simulink model "dcmotor_data"  (R2015a)
settings: Solver=ode23t  StartTime=0.0  StopTime=10.0  RelTol=1e-3  AbsTol=1e-3
libraries: fl_lib x104, nesl_utility x3, elec_lib x1
settings Model: Creator=sseshadr  LastModifiedBy=sseshadr
settings SimscapeCC: SimscapeLogType=all  SimscapeLogOpenViewer=on  SimscapeLogLimitData=off  SimscapeLogDataHistory=10000

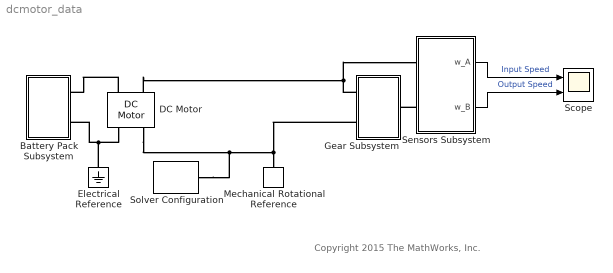
== system dcmotor_data ==
  note: Copyright 2015 The MathWorks, Inc.
  Battery Pack Subsystem : Subsystem
  DC Motor : elec_lib/Actuators & Drivers/Rotational Actuators/DC Motor  parameterization=1  Ra=0.0093 Ohm  La=172 uH  emf_or_torque=1  Kv=0.19 V/rpm  Ki=6.876e-4 N*m/A  T_stall=2.4e-4 N*m  w_max=1.91e+4 rpm  w_rated=1.5e+4 rpm  P_rated=0.08 W  V_rated=1.5 V  J=0.01 g*cm^2  lam_param=1  lam=0 N*m/(rad/s)  i_noload=0 A  V_i_noload=1.5 V  speed0=10 rad/s  alpha=0.00393 1/K  Tmeas=25 C  thermal_mass=100 J/K  initial_temperature=25 C
  Electrical Reference : fl_lib/Electrical/Electrical Elements/Electrical Reference
  Gear Subsystem : Subsystem
  Mechanical Rotational Reference : fl_lib/Mechanical/Rotational Elements/Mechanical Rotational Reference
  Scope : Scope  NumInputPorts=2
      settings: YMin=-5~-5  YMax=5~5
  Sensors Subsystem : Subsystem
  Solver Configuration : nesl_utility/Solver Configuration  PhysicalDomain=network_engine_domain  SubClassName=solver  LeftPortType=input  RightPortType=generic  Accelerate=off  Tones=[]  Harmonics=[]  SimulateNoise=off  Profile=off  UseLocalSampling=off  EnableSwitchedLinearOptims=on  FrequencyDomain=off  UseCCode=off  RelTol=0.001  AbsTol=1e-06  MinStep=1e-09  ToWorkspace=off  RevertToSquareIcSolve=off  NumHomotopyIterations=100  DoDC=off  ResidualTolerance=1e-09  UseLocalSolver=off  LocalSolverChoice=NE_BACKWARD_EULER_ADVANCER  LocalSolverSampleTime=0.001  DoFixedCost=off  MaxNonlinIter=3  MaxModeIter=2  LinearAlgebra=Sparse  DelaysMemoryBudget=1024  AutomaticFiltering=on  FilteringTimeConstant=0.001
  wires:
  Sensors Subsystem/1(w_A) -> Scope/1  "Input Speed"
  Sensors Subsystem/2(w_B) -> Scope/2  "Output Speed"
  connections:
  Solver Configuration/RConn1 -- DC Motor/RConn2 -- Gear Subsystem/LConn2 -- Mechanical Rotational Reference/LConn1
  Gear Subsystem/LConn1 -- DC Motor/LConn2 -- Sensors Subsystem/LConn1
  Sensors Subsystem/LConn2 -- Gear Subsystem/RConn1
  DC Motor/LConn1 -- Battery Pack Subsystem/RConn1
  DC Motor/RConn1 -- Electrical Reference/LConn1 -- Battery Pack Subsystem/RConn2

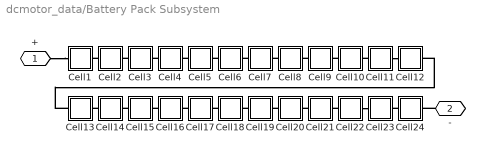
== system dcmotor_data/Battery Pack Subsystem ==
  Cell1 : Subsystem
  Cell10 : Subsystem
  Cell11 : Subsystem
  Cell12 : Subsystem
  Cell13 : Subsystem
  Cell14 : Subsystem
  Cell15 : Subsystem
  Cell16 : Subsystem
  Cell17 : Subsystem
  Cell18 : Subsystem
  Cell19 : Subsystem
  Cell2 : Subsystem
  Cell20 : Subsystem
  Cell21 : Subsystem
  Cell22 : Subsystem
  Cell23 : Subsystem
  Cell24 : Subsystem
  Cell3 : Subsystem
  Cell4 : Subsystem
  Cell5 : Subsystem
  Cell6 : Subsystem
  Cell7 : Subsystem
  Cell8 : Subsystem
  Cell9 : Subsystem
  + : PMIOPort  Port=1  Side=Right
  - : PMIOPort  Port=2  Side=Right
  connections:
  +/RConn1 -- Cell1/LConn1
  Cell2/LConn1 -- Cell1/RConn1
  Cell3/LConn1 -- Cell2/RConn1
  Cell4/LConn1 -- Cell3/RConn1
  Cell5/LConn1 -- Cell4/RConn1
  Cell6/LConn1 -- Cell5/RConn1
  Cell7/LConn1 -- Cell6/RConn1
  Cell8/LConn1 -- Cell7/RConn1
  Cell9/LConn1 -- Cell8/RConn1
  Cell10/LConn1 -- Cell9/RConn1
  Cell11/LConn1 -- Cell10/RConn1
  Cell13/LConn1 -- Cell12/RConn1
  Cell14/LConn1 -- Cell13/RConn1
  Cell15/LConn1 -- Cell14/RConn1
  Cell16/LConn1 -- Cell15/RConn1
  Cell17/LConn1 -- Cell16/RConn1
  Cell18/LConn1 -- Cell17/RConn1
  Cell19/LConn1 -- Cell18/RConn1
  Cell20/LConn1 -- Cell19/RConn1
  Cell21/LConn1 -- Cell20/RConn1
  Cell22/LConn1 -- Cell21/RConn1
  Cell24/LConn1 -- Cell23/RConn1
  -/RConn1 -- Cell24/RConn1
  Cell11/RConn1 -- Cell12/LConn1
  Cell22/RConn1 -- Cell23/LConn1

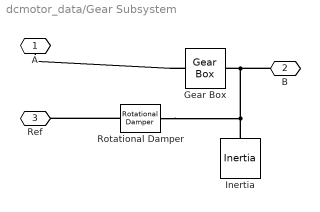
== system dcmotor_data/Gear Subsystem ==
  Gear Box : fl_lib/Mechanical/Mechanisms/Gear Box  ratio=2  t_in_specify=off  t_in_priority=High  t_in=0 N*m  t_out_specify=off  t_out_priority=High  t_out=0 N*m
  Inertia : fl_lib/Mechanical/Rotational Elements/Inertia  inertia=0.01 kg*m^2  w_specify=on  w_priority=Low  w=10 rad/s  t_specify=off  t_priority=High  t=0 N*m
  Rotational Damper : fl_lib/Mechanical/Rotational Elements/Rotational Damper  D=0.001 N*m/(rad/s)  w_specify=off  w_priority=High  w=0 rad/s  t_specify=off  t_priority=High  t=0 N*m
  A : PMIOPort  Port=1  Side=Left
  B : PMIOPort  Port=2  Side=Right
  Ref : PMIOPort  Port=3  Side=Left
  connections:
  Inertia/LConn1 -- Rotational Damper/LConn1 -- B/RConn1 -- Gear Box/RConn1
  Rotational Damper/RConn1 -- Ref/RConn1
  Gear Box/LConn1 -- A/RConn1

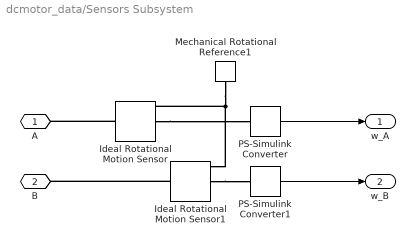
== system dcmotor_data/Sensors Subsystem ==
  Ideal Rotational Motion Sensor : fl_lib/Mechanical/Mechanical Sensors/Ideal Rotational Motion Sensor  offset=0 rad
  Ideal Rotational Motion Sensor1 : fl_lib/Mechanical/Mechanical Sensors/Ideal Rotational Motion Sensor  offset=0 rad
  Mechanical Rotational Reference1 : fl_lib/Mechanical/Rotational Elements/Mechanical Rotational Reference
  PS-Simulink Converter : nesl_utility/PS-Simulink Converter  PhysicalDomain=network_engine_domain  SubClassName=ps_output  LeftPortType=input  RightPortType=output  PseudoPeriodic=off  Frequencies=[]  Unit=1  AffineConversion=off
  PS-Simulink Converter1 : nesl_utility/PS-Simulink Converter  PhysicalDomain=network_engine_domain  SubClassName=ps_output  LeftPortType=input  RightPortType=output  PseudoPeriodic=off  Frequencies=[]  Unit=1  AffineConversion=off
  A : PMIOPort  Port=1  Side=Left
  B : PMIOPort  Port=2  Side=Left
  w_A : Outport
  w_B : Outport  Port=2
  wires:
  PS-Simulink Converter1/1 -> w_B/1
  PS-Simulink Converter/1 -> w_A/1
  connections:
  Ideal Rotational Motion Sensor/LConn1 -- A/RConn1
  Ideal Rotational Motion Sensor1/RConn2 -- PS-Simulink Converter1/LConn1
  Ideal Rotational Motion Sensor/RConn2 -- PS-Simulink Converter/LConn1
  Mechanical Rotational Reference1/LConn1 -- Ideal Rotational Motion Sensor/RConn1 -- Ideal Rotational Motion Sensor1/RConn1
  Ideal Rotational Motion Sensor1/LConn1 -- B/RConn1

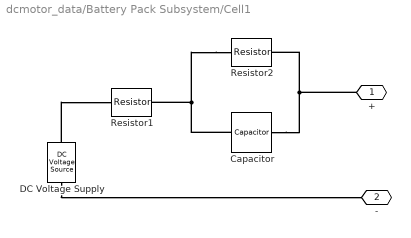
== system dcmotor_data/Battery Pack Subsystem/Cell1 ==
  Capacitor : fl_lib/Electrical/Electrical Elements/Capacitor  c=1e-3 F  r=1e-6 Ohm  g=0 1/Ohm  i_specify=off  i_priority=High  i=0 A  v_specify=off  v_priority=High  v=0 V  vc_specify=on  vc_priority=High  vc=0 V
  DC Voltage Supply : fl_lib/Electrical/Electrical Sources/DC Voltage Source  v0=4.2 V
  Resistor1 : fl_lib/Electrical/Electrical Elements/Resistor  R=0.07 Ohm  i_specify=off  i_priority=High  i=0 A  v_specify=off  v_priority=High  v=0 V
  Resistor2 : fl_lib/Electrical/Electrical Elements/Resistor  R=0.05 Ohm  i_specify=off  i_priority=High  i=0 A  v_specify=off  v_priority=High  v=0 V
  + : PMIOPort  Port=1  Side=Left
  - : PMIOPort  Port=2  Side=Right
  connections:
  Resistor2/LConn1 -- Capacitor/LConn1 -- Resistor1/RConn1
  DC Voltage Supply/RConn1 -- -/RConn1
  Resistor2/RConn1 -- +/RConn1 -- Capacitor/RConn1
  DC Voltage Supply/LConn1 -- Resistor1/LConn1

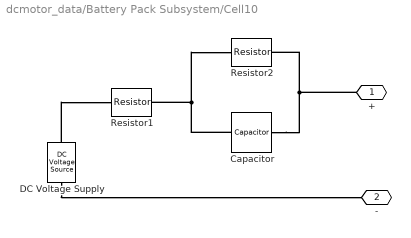
== system dcmotor_data/Battery Pack Subsystem/Cell10 ==
  Capacitor : fl_lib/Electrical/Electrical Elements/Capacitor  c=1e-3 F  r=1e-6 Ohm  g=0 1/Ohm  i_specify=off  i_priority=High  i=0 A  v_specify=off  v_priority=High  v=0 V  vc_specify=on  vc_priority=High  vc=0 V
  DC Voltage Supply : fl_lib/Electrical/Electrical Sources/DC Voltage Source  v0=4.2 V
  Resistor1 : fl_lib/Electrical/Electrical Elements/Resistor  R=0.07 Ohm  i_specify=off  i_priority=High  i=0 A  v_specify=off  v_priority=High  v=0 V
  Resistor2 : fl_lib/Electrical/Electrical Elements/Resistor  R=0.05 Ohm  i_specify=off  i_priority=High  i=0 A  v_specify=off  v_priority=High  v=0 V
  + : PMIOPort  Port=1  Side=Left
  - : PMIOPort  Port=2  Side=Right
  connections:
  DC Voltage Supply/LConn1 -- Resistor1/LConn1
  +/RConn1 -- Capacitor/RConn1 -- Resistor2/RConn1
  DC Voltage Supply/RConn1 -- -/RConn1
  Resistor1/RConn1 -- Capacitor/LConn1 -- Resistor2/LConn1

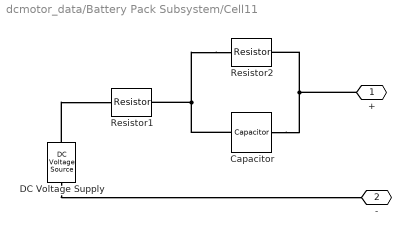
== system dcmotor_data/Battery Pack Subsystem/Cell11 ==
  Capacitor : fl_lib/Electrical/Electrical Elements/Capacitor  c=1e-3 F  r=1e-6 Ohm  g=0 1/Ohm  i_specify=off  i_priority=High  i=0 A  v_specify=off  v_priority=High  v=0 V  vc_specify=on  vc_priority=High  vc=0 V
  DC Voltage Supply : fl_lib/Electrical/Electrical Sources/DC Voltage Source  v0=4.2 V
  Resistor1 : fl_lib/Electrical/Electrical Elements/Resistor  R=0.07 Ohm  i_specify=off  i_priority=High  i=0 A  v_specify=off  v_priority=High  v=0 V
  Resistor2 : fl_lib/Electrical/Electrical Elements/Resistor  R=0.05 Ohm  i_specify=off  i_priority=High  i=0 A  v_specify=off  v_priority=High  v=0 V
  + : PMIOPort  Port=1  Side=Left
  - : PMIOPort  Port=2  Side=Right
  connections:
  Resistor2/LConn1 -- Capacitor/LConn1 -- Resistor1/RConn1
  DC Voltage Supply/RConn1 -- -/RConn1
  Resistor2/RConn1 -- Capacitor/RConn1 -- +/RConn1
  DC Voltage Supply/LConn1 -- Resistor1/LConn1

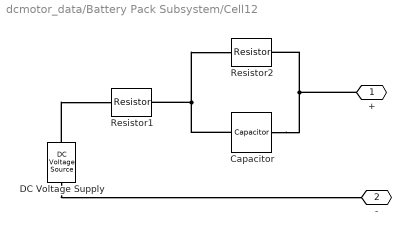
== system dcmotor_data/Battery Pack Subsystem/Cell12 ==
  Capacitor : fl_lib/Electrical/Electrical Elements/Capacitor  c=1e-3 F  r=1e-6 Ohm  g=0 1/Ohm  i_specify=off  i_priority=High  i=0 A  v_specify=off  v_priority=High  v=0 V  vc_specify=on  vc_priority=High  vc=0 V
  DC Voltage Supply : fl_lib/Electrical/Electrical Sources/DC Voltage Source  v0=4.2 V
  Resistor1 : fl_lib/Electrical/Electrical Elements/Resistor  R=0.07 Ohm  i_specify=off  i_priority=High  i=0 A  v_specify=off  v_priority=High  v=0 V
  Resistor2 : fl_lib/Electrical/Electrical Elements/Resistor  R=0.05 Ohm  i_specify=off  i_priority=High  i=0 A  v_specify=off  v_priority=High  v=0 V
  + : PMIOPort  Port=1  Side=Left
  - : PMIOPort  Port=2  Side=Right
  connections:
  DC Voltage Supply/LConn1 -- Resistor1/LConn1
  +/RConn1 -- Capacitor/RConn1 -- Resistor2/RConn1
  DC Voltage Supply/RConn1 -- -/RConn1
  Resistor1/RConn1 -- Capacitor/LConn1 -- Resistor2/LConn1

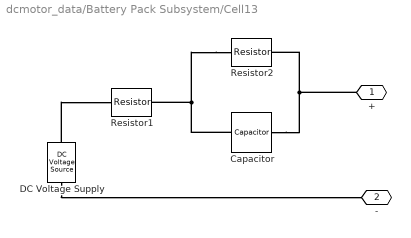
== system dcmotor_data/Battery Pack Subsystem/Cell13 ==
  Capacitor : fl_lib/Electrical/Electrical Elements/Capacitor  c=1e-3 F  r=1e-6 Ohm  g=0 1/Ohm  i_specify=off  i_priority=High  i=0 A  v_specify=off  v_priority=High  v=0 V  vc_specify=on  vc_priority=High  vc=0 V
  DC Voltage Supply : fl_lib/Electrical/Electrical Sources/DC Voltage Source  v0=4.2 V
  Resistor1 : fl_lib/Electrical/Electrical Elements/Resistor  R=0.07 Ohm  i_specify=off  i_priority=High  i=0 A  v_specify=off  v_priority=High  v=0 V
  Resistor2 : fl_lib/Electrical/Electrical Elements/Resistor  R=0.05 Ohm  i_specify=off  i_priority=High  i=0 A  v_specify=off  v_priority=High  v=0 V
  + : PMIOPort  Port=1  Side=Left
  - : PMIOPort  Port=2  Side=Right
  connections:
  Resistor2/LConn1 -- Capacitor/LConn1 -- Resistor1/RConn1
  DC Voltage Supply/RConn1 -- -/RConn1
  Resistor2/RConn1 -- Capacitor/RConn1 -- +/RConn1
  DC Voltage Supply/LConn1 -- Resistor1/LConn1

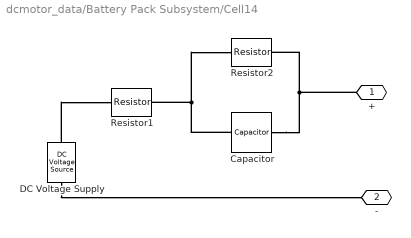
== system dcmotor_data/Battery Pack Subsystem/Cell14 ==
  Capacitor : fl_lib/Electrical/Electrical Elements/Capacitor  c=1e-3 F  r=1e-6 Ohm  g=0 1/Ohm  i_specify=off  i_priority=High  i=0 A  v_specify=off  v_priority=High  v=0 V  vc_specify=on  vc_priority=High  vc=0 V
  DC Voltage Supply : fl_lib/Electrical/Electrical Sources/DC Voltage Source  v0=4.2 V
  Resistor1 : fl_lib/Electrical/Electrical Elements/Resistor  R=0.07 Ohm  i_specify=off  i_priority=High  i=0 A  v_specify=off  v_priority=High  v=0 V
  Resistor2 : fl_lib/Electrical/Electrical Elements/Resistor  R=0.05 Ohm  i_specify=off  i_priority=High  i=0 A  v_specify=off  v_priority=High  v=0 V
  + : PMIOPort  Port=1  Side=Left
  - : PMIOPort  Port=2  Side=Right
  connections:
  DC Voltage Supply/LConn1 -- Resistor1/LConn1
  +/RConn1 -- Capacitor/RConn1 -- Resistor2/RConn1
  DC Voltage Supply/RConn1 -- -/RConn1
  Resistor1/RConn1 -- Capacitor/LConn1 -- Resistor2/LConn1

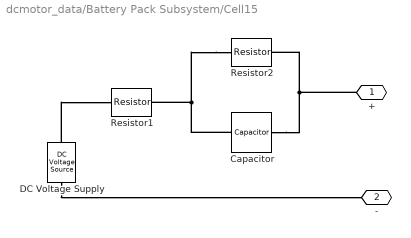
== system dcmotor_data/Battery Pack Subsystem/Cell15 ==
  Capacitor : fl_lib/Electrical/Electrical Elements/Capacitor  c=1e-3 F  r=1e-6 Ohm  g=0 1/Ohm  i_specify=off  i_priority=High  i=0 A  v_specify=off  v_priority=High  v=0 V  vc_specify=on  vc_priority=High  vc=0 V
  DC Voltage Supply : fl_lib/Electrical/Electrical Sources/DC Voltage Source  v0=4.2 V
  Resistor1 : fl_lib/Electrical/Electrical Elements/Resistor  R=0.07 Ohm  i_specify=off  i_priority=High  i=0 A  v_specify=off  v_priority=High  v=0 V
  Resistor2 : fl_lib/Electrical/Electrical Elements/Resistor  R=0.05 Ohm  i_specify=off  i_priority=High  i=0 A  v_specify=off  v_priority=High  v=0 V
  + : PMIOPort  Port=1  Side=Left
  - : PMIOPort  Port=2  Side=Right
  connections:
  Resistor2/LConn1 -- Capacitor/LConn1 -- Resistor1/RConn1
  DC Voltage Supply/RConn1 -- -/RConn1
  Resistor2/RConn1 -- Capacitor/RConn1 -- +/RConn1
  DC Voltage Supply/LConn1 -- Resistor1/LConn1

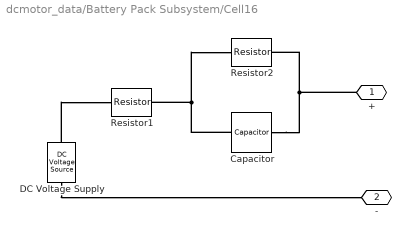
== system dcmotor_data/Battery Pack Subsystem/Cell16 ==
  Capacitor : fl_lib/Electrical/Electrical Elements/Capacitor  c=1e-3 F  r=1e-6 Ohm  g=0 1/Ohm  i_specify=off  i_priority=High  i=0 A  v_specify=off  v_priority=High  v=0 V  vc_specify=on  vc_priority=High  vc=0 V
  DC Voltage Supply : fl_lib/Electrical/Electrical Sources/DC Voltage Source  v0=4.2 V
  Resistor1 : fl_lib/Electrical/Electrical Elements/Resistor  R=0.07 Ohm  i_specify=off  i_priority=High  i=0 A  v_specify=off  v_priority=High  v=0 V
  Resistor2 : fl_lib/Electrical/Electrical Elements/Resistor  R=0.05 Ohm  i_specify=off  i_priority=High  i=0 A  v_specify=off  v_priority=High  v=0 V
  + : PMIOPort  Port=1  Side=Left
  - : PMIOPort  Port=2  Side=Right
  connections:
  DC Voltage Supply/LConn1 -- Resistor1/LConn1
  +/RConn1 -- Capacitor/RConn1 -- Resistor2/RConn1
  DC Voltage Supply/RConn1 -- -/RConn1
  Resistor1/RConn1 -- Capacitor/LConn1 -- Resistor2/LConn1

== system dcmotor_data/Battery Pack Subsystem/Cell17 ==
  Capacitor : fl_lib/Electrical/Electrical Elements/Capacitor  c=1e-3 F  r=1e-6 Ohm  g=0 1/Ohm  i_specify=off  i_priority=High  i=0 A  v_specify=off  v_priority=High  v=0 V  vc_specify=on  vc_priority=High  vc=0 V
  DC Voltage Supply : fl_lib/Electrical/Electrical Sources/DC Voltage Source  v0=4.2 V
  Resistor1 : fl_lib/Electrical/Electrical Elements/Resistor  R=0.07 Ohm  i_specify=off  i_priority=High  i=0 A  v_specify=off  v_priority=High  v=0 V
  Resistor2 : fl_lib/Electrical/Electrical Elements/Resistor  R=0.05 Ohm  i_specify=off  i_priority=High  i=0 A  v_specify=off  v_priority=High  v=0 V
  + : PMIOPort  Port=1  Side=Left
  - : PMIOPort  Port=2  Side=Right
  connections:
  Resistor2/LConn1 -- Capacitor/LConn1 -- Resistor1/RConn1
  DC Voltage Supply/RConn1 -- -/RConn1
  Resistor2/RConn1 -- Capacitor/RConn1 -- +/RConn1
  DC Voltage Supply/LConn1 -- Resistor1/LConn1

== system dcmotor_data/Battery Pack Subsystem/Cell18 ==
  Capacitor : fl_lib/Electrical/Electrical Elements/Capacitor  c=1e-3 F  r=1e-6 Ohm  g=0 1/Ohm  i_specify=off  i_priority=High  i=0 A  v_specify=off  v_priority=High  v=0 V  vc_specify=on  vc_priority=High  vc=0 V
  DC Voltage Supply : fl_lib/Electrical/Electrical Sources/DC Voltage Source  v0=4.2 V
  Resistor1 : fl_lib/Electrical/Electrical Elements/Resistor  R=0.07 Ohm  i_specify=off  i_priority=High  i=0 A  v_specify=off  v_priority=High  v=0 V
  Resistor2 : fl_lib/Electrical/Electrical Elements/Resistor  R=0.05 Ohm  i_specify=off  i_priority=High  i=0 A  v_specify=off  v_priority=High  v=0 V
  + : PMIOPort  Port=1  Side=Left
  - : PMIOPort  Port=2  Side=Right
  connections:
  DC Voltage Supply/LConn1 -- Resistor1/LConn1
  +/RConn1 -- Capacitor/RConn1 -- Resistor2/RConn1
  DC Voltage Supply/RConn1 -- -/RConn1
  Resistor1/RConn1 -- Capacitor/LConn1 -- Resistor2/LConn1

== system dcmotor_data/Battery Pack Subsystem/Cell19 ==
  Capacitor : fl_lib/Electrical/Electrical Elements/Capacitor  c=1e-3 F  r=1e-6 Ohm  g=0 1/Ohm  i_specify=off  i_priority=High  i=0 A  v_specify=off  v_priority=High  v=0 V  vc_specify=on  vc_priority=High  vc=0 V
  DC Voltage Supply : fl_lib/Electrical/Electrical Sources/DC Voltage Source  v0=4.2 V
  Resistor1 : fl_lib/Electrical/Electrical Elements/Resistor  R=0.07 Ohm  i_specify=off  i_priority=High  i=0 A  v_specify=off  v_priority=High  v=0 V
  Resistor2 : fl_lib/Electrical/Electrical Elements/Resistor  R=0.05 Ohm  i_specify=off  i_priority=High  i=0 A  v_specify=off  v_priority=High  v=0 V
  + : PMIOPort  Port=1  Side=Left
  - : PMIOPort  Port=2  Side=Right
  connections:
  Resistor2/LConn1 -- Capacitor/LConn1 -- Resistor1/RConn1
  DC Voltage Supply/RConn1 -- -/RConn1
  Resistor2/RConn1 -- Capacitor/RConn1 -- +/RConn1
  DC Voltage Supply/LConn1 -- Resistor1/LConn1

== system dcmotor_data/Battery Pack Subsystem/Cell2 ==
  Capacitor : fl_lib/Electrical/Electrical Elements/Capacitor  c=1e-3 F  r=1e-6 Ohm  g=0 1/Ohm  i_specify=off  i_priority=High  i=0 A  v_specify=off  v_priority=High  v=0 V  vc_specify=on  vc_priority=High  vc=0 V
  DC Voltage Supply : fl_lib/Electrical/Electrical Sources/DC Voltage Source  v0=4.2 V
  Resistor1 : fl_lib/Electrical/Electrical Elements/Resistor  R=0.07 Ohm  i_specify=off  i_priority=High  i=0 A  v_specify=off  v_priority=High  v=0 V
  Resistor2 : fl_lib/Electrical/Electrical Elements/Resistor  R=0.05 Ohm  i_specify=off  i_priority=High  i=0 A  v_specify=off  v_priority=High  v=0 V
  + : PMIOPort  Port=1  Side=Left
  - : PMIOPort  Port=2  Side=Right
  connections:
  DC Voltage Supply/LConn1 -- Resistor1/LConn1
  +/RConn1 -- Capacitor/RConn1 -- Resistor2/RConn1
  DC Voltage Supply/RConn1 -- -/RConn1
  Resistor1/RConn1 -- Capacitor/LConn1 -- Resistor2/LConn1

== system dcmotor_data/Battery Pack Subsystem/Cell20 ==
  Capacitor : fl_lib/Electrical/Electrical Elements/Capacitor  c=1e-3 F  r=1e-6 Ohm  g=0 1/Ohm  i_specify=off  i_priority=High  i=0 A  v_specify=off  v_priority=High  v=0 V  vc_specify=on  vc_priority=High  vc=0 V
  DC Voltage Supply : fl_lib/Electrical/Electrical Sources/DC Voltage Source  v0=4.2 V
  Resistor1 : fl_lib/Electrical/Electrical Elements/Resistor  R=0.07 Ohm  i_specify=off  i_priority=High  i=0 A  v_specify=off  v_priority=High  v=0 V
  Resistor2 : fl_lib/Electrical/Electrical Elements/Resistor  R=0.05 Ohm  i_specify=off  i_priority=High  i=0 A  v_specify=off  v_priority=High  v=0 V
  + : PMIOPort  Port=1  Side=Left
  - : PMIOPort  Port=2  Side=Right
  connections:
  DC Voltage Supply/LConn1 -- Resistor1/LConn1
  +/RConn1 -- Capacitor/RConn1 -- Resistor2/RConn1
  DC Voltage Supply/RConn1 -- -/RConn1
  Resistor1/RConn1 -- Capacitor/LConn1 -- Resistor2/LConn1

== system dcmotor_data/Battery Pack Subsystem/Cell21 ==
  Capacitor : fl_lib/Electrical/Electrical Elements/Capacitor  c=1e-3 F  r=1e-6 Ohm  g=0 1/Ohm  i_specify=off  i_priority=High  i=0 A  v_specify=off  v_priority=High  v=0 V  vc_specify=on  vc_priority=High  vc=0 V
  DC Voltage Supply : fl_lib/Electrical/Electrical Sources/DC Voltage Source  v0=4.2 V
  Resistor1 : fl_lib/Electrical/Electrical Elements/Resistor  R=0.07 Ohm  i_specify=off  i_priority=High  i=0 A  v_specify=off  v_priority=High  v=0 V
  Resistor2 : fl_lib/Electrical/Electrical Elements/Resistor  R=0.05 Ohm  i_specify=off  i_priority=High  i=0 A  v_specify=off  v_priority=High  v=0 V
  + : PMIOPort  Port=1  Side=Left
  - : PMIOPort  Port=2  Side=Right
  connections:
  Resistor2/LConn1 -- Capacitor/LConn1 -- Resistor1/RConn1
  DC Voltage Supply/RConn1 -- -/RConn1
  Resistor2/RConn1 -- Capacitor/RConn1 -- +/RConn1
  DC Voltage Supply/LConn1 -- Resistor1/LConn1

== system dcmotor_data/Battery Pack Subsystem/Cell22 ==
  Capacitor : fl_lib/Electrical/Electrical Elements/Capacitor  c=1e-3 F  r=1e-6 Ohm  g=0 1/Ohm  i_specify=off  i_priority=High  i=0 A  v_specify=off  v_priority=High  v=0 V  vc_specify=on  vc_priority=High  vc=0 V
  DC Voltage Supply : fl_lib/Electrical/Electrical Sources/DC Voltage Source  v0=4.2 V
  Resistor1 : fl_lib/Electrical/Electrical Elements/Resistor  R=0.07 Ohm  i_specify=off  i_priority=High  i=0 A  v_specify=off  v_priority=High  v=0 V
  Resistor2 : fl_lib/Electrical/Electrical Elements/Resistor  R=0.05 Ohm  i_specify=off  i_priority=High  i=0 A  v_specify=off  v_priority=High  v=0 V
  + : PMIOPort  Port=1  Side=Left
  - : PMIOPort  Port=2  Side=Right
  connections:
  DC Voltage Supply/LConn1 -- Resistor1/LConn1
  +/RConn1 -- Capacitor/RConn1 -- Resistor2/RConn1
  DC Voltage Supply/RConn1 -- -/RConn1
  Resistor1/RConn1 -- Capacitor/LConn1 -- Resistor2/LConn1

== system dcmotor_data/Battery Pack Subsystem/Cell23 ==
  Capacitor : fl_lib/Electrical/Electrical Elements/Capacitor  c=1e-3 F  r=1e-6 Ohm  g=0 1/Ohm  i_specify=off  i_priority=High  i=0 A  v_specify=off  v_priority=High  v=0 V  vc_specify=on  vc_priority=High  vc=0 V
  DC Voltage Supply : fl_lib/Electrical/Electrical Sources/DC Voltage Source  v0=4.2 V
  Resistor1 : fl_lib/Electrical/Electrical Elements/Resistor  R=0.07 Ohm  i_specify=off  i_priority=High  i=0 A  v_specify=off  v_priority=High  v=0 V
  Resistor2 : fl_lib/Electrical/Electrical Elements/Resistor  R=0.05 Ohm  i_specify=off  i_priority=High  i=0 A  v_specify=off  v_priority=High  v=0 V
  + : PMIOPort  Port=1  Side=Left
  - : PMIOPort  Port=2  Side=Right
  connections:
  Resistor2/LConn1 -- Capacitor/LConn1 -- Resistor1/RConn1
  DC Voltage Supply/RConn1 -- -/RConn1
  Resistor2/RConn1 -- Capacitor/RConn1 -- +/RConn1
  DC Voltage Supply/LConn1 -- Resistor1/LConn1

== system dcmotor_data/Battery Pack Subsystem/Cell24 ==
  Capacitor : fl_lib/Electrical/Electrical Elements/Capacitor  c=1e-3 F  r=1e-6 Ohm  g=0 1/Ohm  i_specify=off  i_priority=High  i=0 A  v_specify=off  v_priority=High  v=0 V  vc_specify=on  vc_priority=High  vc=0 V
  DC Voltage Supply : fl_lib/Electrical/Electrical Sources/DC Voltage Source  v0=4.2 V
  Resistor1 : fl_lib/Electrical/Electrical Elements/Resistor  R=0.07 Ohm  i_specify=off  i_priority=High  i=0 A  v_specify=off  v_priority=High  v=0 V
  Resistor2 : fl_lib/Electrical/Electrical Elements/Resistor  R=0.05 Ohm  i_specify=off  i_priority=High  i=0 A  v_specify=off  v_priority=High  v=0 V
  + : PMIOPort  Port=1  Side=Left
  - : PMIOPort  Port=2  Side=Right
  connections:
  DC Voltage Supply/LConn1 -- Resistor1/LConn1
  +/RConn1 -- Capacitor/RConn1 -- Resistor2/RConn1
  DC Voltage Supply/RConn1 -- -/RConn1
  Resistor1/RConn1 -- Capacitor/LConn1 -- Resistor2/LConn1

== system dcmotor_data/Battery Pack Subsystem/Cell3 ==
  Capacitor : fl_lib/Electrical/Electrical Elements/Capacitor  c=1e-3 F  r=1e-6 Ohm  g=0 1/Ohm  i_specify=off  i_priority=High  i=0 A  v_specify=off  v_priority=High  v=0 V  vc_specify=on  vc_priority=High  vc=0 V
  DC Voltage Supply : fl_lib/Electrical/Electrical Sources/DC Voltage Source  v0=4.2 V
  Resistor1 : fl_lib/Electrical/Electrical Elements/Resistor  R=0.07 Ohm  i_specify=off  i_priority=High  i=0 A  v_specify=off  v_priority=High  v=0 V
  Resistor2 : fl_lib/Electrical/Electrical Elements/Resistor  R=0.05 Ohm  i_specify=off  i_priority=High  i=0 A  v_specify=off  v_priority=High  v=0 V
  + : PMIOPort  Port=1  Side=Left
  - : PMIOPort  Port=2  Side=Right
  connections:
  Resistor2/LConn1 -- Capacitor/LConn1 -- Resistor1/RConn1
  DC Voltage Supply/RConn1 -- -/RConn1
  Resistor2/RConn1 -- Capacitor/RConn1 -- +/RConn1
  DC Voltage Supply/LConn1 -- Resistor1/LConn1

== system dcmotor_data/Battery Pack Subsystem/Cell4 ==
  Capacitor : fl_lib/Electrical/Electrical Elements/Capacitor  c=1e-3 F  r=1e-6 Ohm  g=0 1/Ohm  i_specify=off  i_priority=High  i=0 A  v_specify=off  v_priority=High  v=0 V  vc_specify=on  vc_priority=High  vc=0 V
  DC Voltage Supply : fl_lib/Electrical/Electrical Sources/DC Voltage Source  v0=4.2 V
  Resistor1 : fl_lib/Electrical/Electrical Elements/Resistor  R=0.07 Ohm  i_specify=off  i_priority=High  i=0 A  v_specify=off  v_priority=High  v=0 V
  Resistor2 : fl_lib/Electrical/Electrical Elements/Resistor  R=0.05 Ohm  i_specify=off  i_priority=High  i=0 A  v_specify=off  v_priority=High  v=0 V
  + : PMIOPort  Port=1  Side=Left
  - : PMIOPort  Port=2  Side=Right
  connections:
  DC Voltage Supply/LConn1 -- Resistor1/LConn1
  +/RConn1 -- Capacitor/RConn1 -- Resistor2/RConn1
  DC Voltage Supply/RConn1 -- -/RConn1
  Resistor1/RConn1 -- Capacitor/LConn1 -- Resistor2/LConn1

== system dcmotor_data/Battery Pack Subsystem/Cell5 ==
  Capacitor : fl_lib/Electrical/Electrical Elements/Capacitor  c=1e-3 F  r=1e-6 Ohm  g=0 1/Ohm  i_specify=off  i_priority=High  i=0 A  v_specify=off  v_priority=High  v=0 V  vc_specify=on  vc_priority=High  vc=0 V
  DC Voltage Supply : fl_lib/Electrical/Electrical Sources/DC Voltage Source  v0=4.2 V
  Resistor1 : fl_lib/Electrical/Electrical Elements/Resistor  R=0.07 Ohm  i_specify=off  i_priority=High  i=0 A  v_specify=off  v_priority=High  v=0 V
  Resistor2 : fl_lib/Electrical/Electrical Elements/Resistor  R=0.05 Ohm  i_specify=off  i_priority=High  i=0 A  v_specify=off  v_priority=High  v=0 V
  + : PMIOPort  Port=1  Side=Left
  - : PMIOPort  Port=2  Side=Right
  connections:
  Resistor2/LConn1 -- Capacitor/LConn1 -- Resistor1/RConn1
  DC Voltage Supply/RConn1 -- -/RConn1
  Resistor2/RConn1 -- Capacitor/RConn1 -- +/RConn1
  DC Voltage Supply/LConn1 -- Resistor1/LConn1

== system dcmotor_data/Battery Pack Subsystem/Cell6 ==
  Capacitor : fl_lib/Electrical/Electrical Elements/Capacitor  c=1e-3 F  r=1e-6 Ohm  g=0 1/Ohm  i_specify=off  i_priority=High  i=0 A  v_specify=off  v_priority=High  v=0 V  vc_specify=on  vc_priority=High  vc=0 V
  DC Voltage Supply : fl_lib/Electrical/Electrical Sources/DC Voltage Source  v0=4.2 V
  Resistor1 : fl_lib/Electrical/Electrical Elements/Resistor  R=0.07 Ohm  i_specify=off  i_priority=High  i=0 A  v_specify=off  v_priority=High  v=0 V
  Resistor2 : fl_lib/Electrical/Electrical Elements/Resistor  R=0.05 Ohm  i_specify=off  i_priority=High  i=0 A  v_specify=off  v_priority=High  v=0 V
  + : PMIOPort  Port=1  Side=Left
  - : PMIOPort  Port=2  Side=Right
  connections:
  DC Voltage Supply/LConn1 -- Resistor1/LConn1
  +/RConn1 -- Capacitor/RConn1 -- Resistor2/RConn1
  DC Voltage Supply/RConn1 -- -/RConn1
  Resistor1/RConn1 -- Capacitor/LConn1 -- Resistor2/LConn1

== system dcmotor_data/Battery Pack Subsystem/Cell7 ==
  Capacitor : fl_lib/Electrical/Electrical Elements/Capacitor  c=1e-3 F  r=1e-6 Ohm  g=0 1/Ohm  i_specify=off  i_priority=High  i=0 A  v_specify=off  v_priority=High  v=0 V  vc_specify=on  vc_priority=High  vc=0 V
  DC Voltage Supply : fl_lib/Electrical/Electrical Sources/DC Voltage Source  v0=4.2 V
  Resistor1 : fl_lib/Electrical/Electrical Elements/Resistor  R=0.07 Ohm  i_specify=off  i_priority=High  i=0 A  v_specify=off  v_priority=High  v=0 V
  Resistor2 : fl_lib/Electrical/Electrical Elements/Resistor  R=0.05 Ohm  i_specify=off  i_priority=High  i=0 A  v_specify=off  v_priority=High  v=0 V
  + : PMIOPort  Port=1  Side=Left
  - : PMIOPort  Port=2  Side=Right
  connections:
  Resistor2/LConn1 -- Capacitor/LConn1 -- Resistor1/RConn1
  DC Voltage Supply/RConn1 -- -/RConn1
  Resistor2/RConn1 -- Capacitor/RConn1 -- +/RConn1
  DC Voltage Supply/LConn1 -- Resistor1/LConn1

== system dcmotor_data/Battery Pack Subsystem/Cell8 ==
  Capacitor : fl_lib/Electrical/Electrical Elements/Capacitor  c=1e-3 F  r=1e-6 Ohm  g=0 1/Ohm  i_specify=off  i_priority=High  i=0 A  v_specify=off  v_priority=High  v=0 V  vc_specify=on  vc_priority=High  vc=0 V
  DC Voltage Supply : fl_lib/Electrical/Electrical Sources/DC Voltage Source  v0=4.2 V
  Resistor1 : fl_lib/Electrical/Electrical Elements/Resistor  R=0.07 Ohm  i_specify=off  i_priority=High  i=0 A  v_specify=off  v_priority=High  v=0 V
  Resistor2 : fl_lib/Electrical/Electrical Elements/Resistor  R=0.05 Ohm  i_specify=off  i_priority=High  i=0 A  v_specify=off  v_priority=High  v=0 V
  + : PMIOPort  Port=1  Side=Left
  - : PMIOPort  Port=2  Side=Right
  connections:
  DC Voltage Supply/LConn1 -- Resistor1/LConn1
  +/RConn1 -- Capacitor/RConn1 -- Resistor2/RConn1
  DC Voltage Supply/RConn1 -- -/RConn1
  Resistor1/RConn1 -- Capacitor/LConn1 -- Resistor2/LConn1

== system dcmotor_data/Battery Pack Subsystem/Cell9 ==
  Capacitor : fl_lib/Electrical/Electrical Elements/Capacitor  c=1e-3 F  r=1e-6 Ohm  g=0 1/Ohm  i_specify=off  i_priority=High  i=0 A  v_specify=off  v_priority=High  v=0 V  vc_specify=on  vc_priority=High  vc=0 V
  DC Voltage Supply : fl_lib/Electrical/Electrical Sources/DC Voltage Source  v0=4.2 V
  Resistor1 : fl_lib/Electrical/Electrical Elements/Resistor  R=0.07 Ohm  i_specify=off  i_priority=High  i=0 A  v_specify=off  v_priority=High  v=0 V
  Resistor2 : fl_lib/Electrical/Electrical Elements/Resistor  R=0.05 Ohm  i_specify=off  i_priority=High  i=0 A  v_specify=off  v_priority=High  v=0 V
  + : PMIOPort  Port=1  Side=Left
  - : PMIOPort  Port=2  Side=Right
  connections:
  Resistor2/LConn1 -- Capacitor/LConn1 -- Resistor1/RConn1
  DC Voltage Supply/RConn1 -- -/RConn1
  Resistor2/RConn1 -- Capacitor/RConn1 -- +/RConn1
  DC Voltage Supply/LConn1 -- Resistor1/LConn1
